simulink model "Torque_Control_ETR07"  (R2017b)
settings: Solver=FixedStepAuto  StartTime=0.0  StopTime=10.0  RelTol=1e-3
libraries: simulink x15
(part 2 of 5)

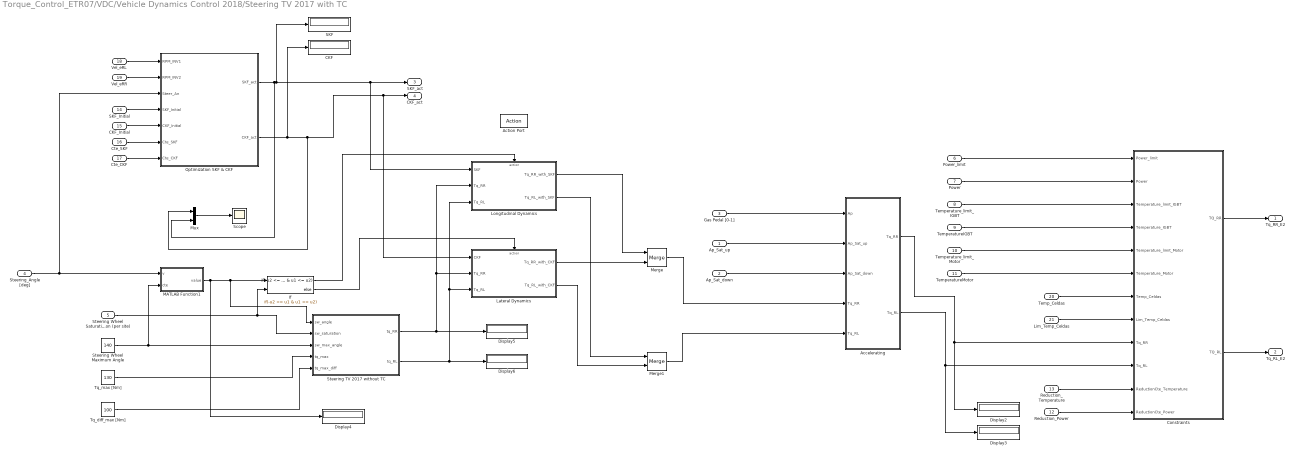
== system Torque_Control_ETR07/VDC/Vehicle Dynamics Control 2018/Steering TV 2017 with TC ==
  "Ap_Sat_up " : Inport
  Ap_Sat_down : Inport  Port=2
  Gas Pedal [0-1] : Inport  Port=3
  Steering_Angle [deg] : Inport  Port=4
  "Steering Wheel Saturation (per site) " : Inport  Port=5
  Power_limit : Inport  Port=6
  Power : Inport  Port=7
  Temperature_limit_IGBT : Inport  Port=8
  TemperatureIGBT : Inport  Port=9
  Temperature_limit_Motor : Inport  Port=10
  TemperatureMotor : Inport  Port=11
  Reduction_Power : Inport  Port=12
  Reduction_Temperature : Inport  Port=13
  SKF_Initial : Inport  Port=14
  CKF_Initial : Inport  Port=15
  Cte_SKF : Inport  Port=16
  Cte_CKF : Inport  Port=17
  Vel_eRL : Inport  Port=18
  Vel_eRR : Inport  Port=19
  Temp_Celdas : Inport  Port=20
  Lim_Temp_Celdas : Inport  Port=21
  Action Port : ActionPort  ActionType=elseif
  Accelerating : Subsystem
  CKF : Display
  Constraints : Subsystem
  Display{2..6} (5 alike) : Display
  If : If  NumInputs=2  IfExpression=-u2 <= u1 & u1 <= u2
  Lateral Dynamics : Subsystem  TreatAsAtomicUnit=on
  Longitudinal Dynamics : Subsystem  TreatAsAtomicUnit=on
  MATLAB Function1 : MATLAB Function  TreatAsAtomicUnit=on
  Merge : Merge
  Merge1 : Merge
  Mux : Mux  Inputs=2
  Optimization SKF & CKF : Subsystem
  SKF : Display
  Scope : Scope
  Steering TV 2017 without TC : MATLAB Function  TreatAsAtomicUnit=on
  Steering Wheel Maximum Angle : Constant  Value=140
  Tq_diff_max [Nm] : Constant  Value=100
  Tq_max [Nm] : Constant  Value=130
  Tq_RR_E2 : Outport
  Tq_RL_E2 : Outport  Port=2
  SKF_act : Outport  Port=3
  CKF_act : Outport  Port=4
  wires:
  Gas Pedal [0-1]/1 -> Accelerating/1(Ap)
  "Ap_Sat_up "/1 -> Accelerating/2("Ap_Sat_up ")
  Ap_Sat_down/1 -> Accelerating/3(Ap_Sat_down)
  Tq_max [Nm]/1 -> Steering TV 2017 without TC/4(tq_max)
  Tq_diff_max [Nm]/1 -> Steering TV 2017 without TC/5(tq_max_diff)
  Steering Wheel Maximum Angle/1 -> Steering TV 2017 without TC/3(sw_max_angle), MATLAB Function1/2(cte)
  "Steering Wheel Saturation (per site) "/1 -> If/2, Steering TV 2017 without TC/2(sw_saturation)
  Steering TV 2017 without TC/1(tq_RR) -> Display5/1, Longitudinal Dynamics/2(Tq_RR), Lateral Dynamics/2(Tq_RR)
  Steering TV 2017 without TC/2(tq_RL) -> Longitudinal Dynamics/3(Tq_RL), Lateral Dynamics/3(Tq_RL), Display6/1
  Power_limit/1 -> Constraints/1(Power_limit)
  Power/1 -> Constraints/2(Power)
  Temperature_limit_IGBT/1 -> Constraints/3(Temperature_limit_IGBT)
  TemperatureIGBT/1 -> Constraints/4(Temperature_IGBT)
  Reduction_Temperature/1 -> Constraints/11(ReductionCte_Temperature)
  Reduction_Power/1 -> Constraints/12(ReductionCte_Power)
  Constraints/1(TQ_RR) -> Tq_RR_E2/1
  Constraints/2(TQ_RL) -> Tq_RL_E2/1
  Accelerating/2(Tq_RL) -> Display3/1, Constraints/10(Tq_RL)
  Accelerating/1("Tq_RR ") -> Display2/1, Constraints/9(Tq_RR)
  MATLAB Function1/1(value) -> Display4/1, Steering TV 2017 without TC/1(sw_angle), If/1
  Temperature_limit_Motor/1 -> Constraints/5(Temperature_limit_Motor)
  TemperatureMotor/1 -> Constraints/6(Temperature_Motor)
  Optimization SKF & CKF/2(CKF_act) -> CKF/1, Mux/1, Lateral Dynamics/1(CKF), CKF_act/1
  SKF_Initial/1 -> Optimization SKF & CKF/4(SKF_Initial)
  Mux/1 -> Scope/1
  Cte_SKF/1 -> Optimization SKF & CKF/6(Cte_SKF)
  Vel_eRL/1 -> Optimization SKF & CKF/1(RPM_INV1)
  Vel_eRR/1 -> Optimization SKF & CKF/2(RPM_INV2)
  Optimization SKF & CKF/1(SKF_act) -> SKF_act/1, Longitudinal Dynamics/1(SKF), SKF/1, Mux/2
  Steering_Angle [deg]/1 -> MATLAB Function1/1(v), Optimization SKF & CKF/3(Steer_An)
  CKF_Initial/1 -> Optimization SKF & CKF/5(CKF_Initial)
  Cte_CKF/1 -> Optimization SKF & CKF/7(Cte_CKF)
  If/1 -> Longitudinal Dynamics/Action
  Lateral Dynamics/2(Tq_RL_with_CKF) -> Merge1/2
  If/2 -> Lateral Dynamics/Action
  Longitudinal Dynamics/2(Tq_RL_with_SKF) -> Merge1/1
  Longitudinal Dynamics/1(Tq_RR_with_SKF) -> Merge/1
  Lateral Dynamics/1(Tq_RR_with_CKF) -> Merge/2
  Merge/1 -> Accelerating/4(Tq_RR)
  Merge1/1 -> Accelerating/5("Tq_RL ")
  Temp_Celdas/1 -> Constraints/7(Temp_Celdas)
  Lim_Temp_Celdas/1 -> Constraints/8(Lim_Temp_Celdas)

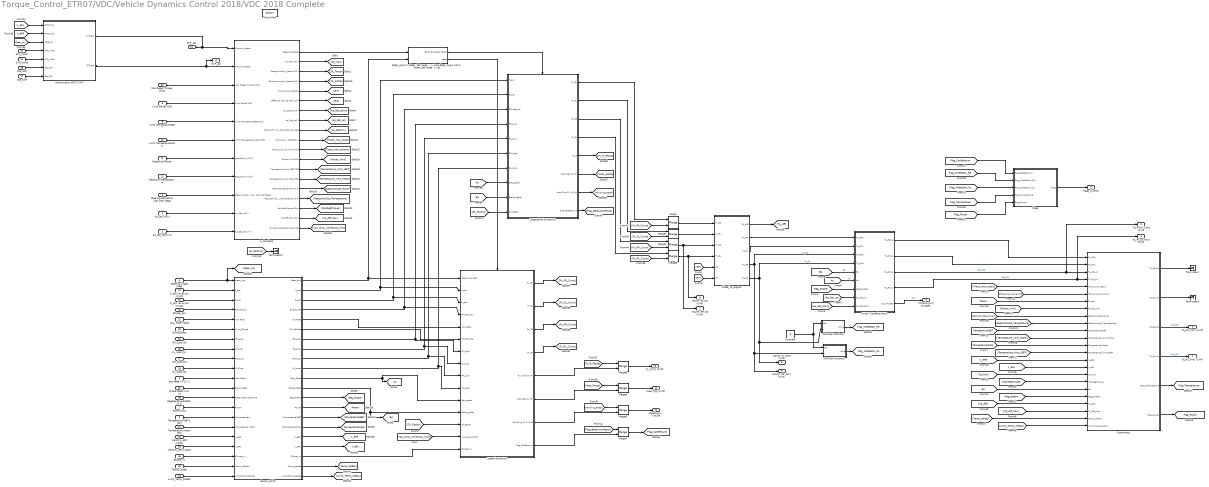
== system Torque_Control_ETR07/VDC/Vehicle Dynamics Control 2018/VDC 2018 Complete ==
  Ap_Sat_Up [-] : Inport
  Ap_Sat_Down [-] : Inport  Port=2
  Gas Pedal (0-1) [-] : Inport  Port=3
  Steering_Angle [deg] : Inport  Port=4
  Steering Saturation (per site) [deg] : Inport  Port=5
  Limit Power [kW] : Inport  Port=6
  Power [kW] : Inport  Port=7
  Limit TemperatureIGBT : Inport  Port=8
  Temperature IGBTs [ºC] : Inport  Port=9
  Limit TemperatureMotor : Inport  Port=10
  Temperature Motor [ºC] : Inport  Port=11
  Reduction Power : Inport  Port=12
  Reduction Temperature : Inport  Port=13
  SKF_Initial : Inport  Port=14
  CKF_Initial : Inport  Port=15
  Cte_SKF : Inport  Port=16
  Cte_CKF : Inport  Port=17
  Velocity_eRL [rad/s] : Inport  Port=18
  Velocity_eRR [rad/s] : Inport  Port=19
  Temp_Celdas : Inport  Port=20
  Limit_Temp_Celdas : Inport  Port=21
  F_acc (ax,ay,az) [m/s2] : Inport  Port=22
  R_acc (ax,ay,az) [m/s2] : Inport  Port=23
  Ellipse_acc : Inport  Port=24
  FR_Susp [N] : Inport  Port=25
  FL_Susp [N] : Inport  Port=26
  RR_Susp [N] : Inport  Port=27
  RL_Susp [N] : Inport  Port=28
  Regenerative Enable [0,1] : Inport  Port=29
  Max Regen Torque [Nm] : Inport  Port=30
  Brake Pedal (0-1) [-] : Inport  Port=31
  Yaw_Rate [rad/s] : Inport  Port=32
  Gyro_Ellipse : Inport  Port=33
  Ellipse_vx : Inport  Port=34
  Action Port : ActionPort  ActionType=then
  Constant : Constant  Value=0
  Constraints : Subsystem
  Driver / CarBehaviours : Subsystem
  Flags : Subsystem
  In_Numbers : Subsystem
  Lateral Dynamics : Subsystem  TreatAsAtomicUnit=on
  Longitudinal Dynamics : Subsystem  TreatAsAtomicUnit=on
  MATLAB Function1 : MATLAB Function  TreatAsAtomicUnit=on
  MATLAB Function2 : MATLAB Function  TreatAsAtomicUnit=on
  Merge{,1..7} (8 alike) : Merge
  Optimization SKF & CKF : Subsystem
  Sensor_DATA : Subsystem
  "Steer_ang is in Steer_Sat range ---> Long Steer_ang is not in Steer_Sat range -> Lat " : If  NumInputs=2  IfExpression=u2>=-u1&u2<=u1
  Terminator : Terminator
  Terminator1 : Terminator
  Terminator2 : Terminator
  Wheel_to_engine : Subsystem
  Tq_RR [Nm] (0,inf) : Outport
  Tq_RL [Nm] (0,inf) : Outport  Port=2
  Tq_RRwc [Nm] (0,inf) : Outport  Port=3
  Tq_RLwc [Nm] (0,inf) : Outport  Port=4
  MaxTq_RR [Nm] (0,inf) : Outport  Port=5
  MaxTq_RL [Nm] (0,inf) : Outport  Port=6
  MaxFx_RR [N] (0,inf) : Outport  Port=7
  MaxFx_RL [N] (0,inf) : Outport  Port=8
  Throttle [0-1] (0-100%) : Outport  Port=9
  Fy_R [N] (0,inf) : Outport  Port=10
  Mass [kg] (0,inf) : Outport  Port=11
  Handling [-] (-inf,inf) : Outport  Port=12
  Flags_[num5] : Outport  Port=13
  SKF_act : Outport  Port=14
  CKF_act : Outport  Port=15
  tag scope: Ap=global, Bp=global, Flag_CarBehavior=global, Flag_Power=global, Flag_Temperature=global, Flag_WheelSpin_RL=global, Flag_WheelSpin_RR=global, Power=global, Reg_enable=global, TemperatureIGBT=global, TemperatureMotor=global, V_eRL=global, V_eRR=global
  wires:
  "Steer_ang is in Steer_Sat range ---> Long Steer_ang is not in Steer_Sat range -> Lat "/1 -> Longitudinal Dynamics/Action
  "Steer_ang is in Steer_Sat range ---> Long Steer_ang is not in Steer_Sat range -> Lat "/2 -> Lateral Dynamics/Action
  Sensor_DATA/10(RL_susp) -> Lateral Dynamics/10(RL_susp), Longitudinal Dynamics/7(RL_susp)
  In_Numbers/3(Straight Kamm_Factor [0-2]) -> [SK_Factor]
  In_Numbers/1(Steer_Sat [deg]) -> "Steer_ang is in Steer_Sat range ---> Long Steer_ang is not in Steer_Sat range -> Lat "/1
  In_Numbers/2(Tq_Max [Nm]) -> [Tq_max]
  Sensor_DATA/11(Gas_Pedal) -> [Ap], Lateral Dynamics/11(Gas_pedal)
  In_Numbers/6(Effective Rolling Radius[m]) -> [Re]
  In_Numbers/5(Transmision_Ratio[-]) -> [RT]
  Sensor_DATA/9(RR_susp) -> Lateral Dynamics/9(RR_susp), Longitudinal Dynamics/6(RR_susp)
  In_Numbers/8(Ap_Sat_up[-]) -> [Ap_Sat_up]
  In_Numbers/7(Ap_Sat_down[-]) -> [Ap_Sat_down]
  Driver / CarBehaviours/3(Tq_RRout) -> Tq_RRwc [Nm] (0,inf)/1, Constraints/3(Tq_RR_wc)  "Teo_RR"
  Sensor_DATA/2(F_acc) -> Lateral Dynamics/2(F_acc), Longitudinal Dynamics/1(F_acc)
  Sensor_DATA/3(R_acc) -> Lateral Dynamics/3(R_acc), Longitudinal Dynamics/2(R_acc)
  Sensor_DATA/12(Brake_Pedal) -> [Bp], Lateral Dynamics/12(Brake_pedal)
  Sensor_DATA/8(FL_susp) -> Lateral Dynamics/8(FL_susp), Longitudinal Dynamics/5(FL_susp)
  Sensor_DATA/13(Reg_Enable) -> [Reg_enable]
  Sensor_DATA/7(FR_susp) -> Lateral Dynamics/7(FR_susp), Longitudinal Dynamics/4(FR_susp)
  Sensor_DATA/1(Steer_ang) -> "Steer_ang is in Steer_Sat range ---> Long Steer_ang is not in Steer_Sat range -> Lat "/2, Lateral Dynamics/1(Steering_Angle)
  Wheel_to_engine/5(Tq_RL) -> Driver / CarBehaviours/4("Tq_RLin "), MaxTq_RL [Nm] (0,inf)/1, MATLAB Function1/2(v)  "Tq_RL"
  [Trans_max_dynamic] -> Constraints/6(Trans_max_dynamic)
  [Power_limit] -> Constraints/8(Power_limit)
  In_Numbers/15(ReductionCte_Power (0-1)) -> [ReductionCte_Power]
  Driver / CarBehaviours/5(out_Throttle) -> Throttle [0-1] (0-100%)/1  "Out"
  Wheel_to_engine/4(Tq_RR) -> Driver / CarBehaviours/3(Tq_RRin), MaxTq_RR [Nm] (0,inf)/1, MATLAB Function2/2(v)  "Tq_RR"
  Wheel_to_engine/3(Tq_FL) -> Driver / CarBehaviours/2(Tq_FLin)
  In_Numbers/11(Trans_max_dynamic [Nm]) -> [Trans_max_dynamic]
  [Reg_enable] -> Driver / CarBehaviours/7(Reg_enable)
  [ReductionCte_Power] -> Constraints/9(ReductionCte_Power)
  [Ap_Sat_up] -> Driver / CarBehaviours/8(Ap_Sat_up)
  In_Numbers/10(Trans_max _static[Nm]) -> [Trans_max_static]
  [Ap] -> Driver / CarBehaviours/6(Ap)  "Ap"
  [Power] -> Constraints/7(Power)
  In_Numbers/12("Power limit [KW] ") -> [Power_limit]
  [Ap_Sat_down] -> Driver / CarBehaviours/9(Ap_Sat_down)
  Driver / CarBehaviours/4(Tq_RLout) -> Tq_RLwc [Nm] (0,inf)/1, Constraints/4("Tq_RL_wc ")  "Teo_RL"
  Driver / CarBehaviours/2("Tq_FLout ") -> Constraints/2(Tq_FLin)
  Steering_Angle [deg]/1 -> [Steer_An], Sensor_DATA/1(Steer_Ang)
  Wheel_to_engine/2(Tq_FR) -> Driver / CarBehaviours/1(Tq_FRin)
  Driver / CarBehaviours/1(Tq_FRout) -> Constraints/1(Tq_FRin)
  [Trans_max_static] -> Constraints/5("Trans_max_static ")
  [Temperature_limit_IGBT] -> Constraints/14(Temperature_limit_IGBT)
  [Bp] -> Constraints/19(Bp)
  Sensor_DATA/18(V_eRL) -> [V_eRL]
  In_Numbers/17(MaxRegTorque [Nm]) -> [MaxRegTorque]
  [TemperatureIGBT] -> Constraints/11(TemperatureIGBT)
  [Reg_enable] -> Constraints/20(Reg_enable)
  In_Numbers/9(Engine+Inverter Performance[-]) -> [ei_Perform]
  [Bp] -> Driver / CarBehaviours/5(Bp)  "Bp"
  [Tq_max] -> Constraints/17(Tq_max)
  RR_Susp [N]/1 -> Sensor_DATA/9(RR_Susp)
  Power [kW]/1 -> Sensor_DATA/14("Power ")
  Sensor_DATA/14(Power) -> [Power]
  Sensor_DATA/17("V_eRR ") -> [V_eRR]
  [V_eRR] -> Constraints/15(V_eRR)
  Regenerative Enable [0,1]/1 -> Sensor_DATA/13(Regenerative Enable)
  Brake Pedal (0-1) [-]/1 -> Sensor_DATA/12(Brake Pedal)
  [V_eRL] -> Constraints/16(V_eRL)
  In_Numbers/13(Temperature limit IGBT [ºC]) -> [Temperature_limit_IGBT]
  FL_Susp [N]/1 -> Sensor_DATA/8(FL_Susp)
  FR_Susp [N]/1 -> Sensor_DATA/7(FR_Susp)
  R_acc (ax,ay,az) [m/s2]/1 -> Sensor_DATA/3(R_Acc)
  F_acc (ax,ay,az) [m/s2]/1 -> Sensor_DATA/2("F_Acc ")
  RL_Susp [N]/1 -> Sensor_DATA/10(RL_Susp)
  Gas Pedal (0-1) [-]/1 -> Sensor_DATA/11(Gas Pedal)
  Temperature IGBTs [ºC]/1 -> Sensor_DATA/15(TemperatureIN)
  Velocity_eRR [rad/s]/1 -> Sensor_DATA/17(V_eRR)
  Velocity_eRL [rad/s]/1 -> Sensor_DATA/18("V_eRL ")
  Constraints/1(Tq_FRout) -> Terminator/1
  Constraints/2("Tq_FLout ") -> Terminator1/1
  In_Numbers/4(Cornering Kamm_Factor [0-2]) -> [CK_Factor]
  [Re] -> Wheel_to_engine/5(Re)
  [RT] -> Wheel_to_engine/6(RT)
  Merge3/1 -> MaxFx_RL [N] (0,inf)/1, Wheel_to_engine/4("Fx_RL ")
  Merge2/1 -> MaxFx_RR [N] (0,inf)/1, Wheel_to_engine/3("Fx_RR ")
  Merge1/1 -> Wheel_to_engine/2("Fx_FL ")
  Max Regen Torque [Nm]/1 -> In_Numbers/3(Max Regen Torque [Nm])
  Limit Power [kW]/1 -> In_Numbers/4(Limit Power [kW])
  Limit TemperatureIGBT/1 -> In_Numbers/5(Limit TemperatureIGBT [ºC])
  Reduction Power/1 -> In_Numbers/7(Reduction_P [0-1])
  [CK_Factor] -> Lateral Dynamics/13(CK_Factor)
  [SK_Factor] -> Longitudinal Dynamics/10(SK_Factor)
  Longitudinal Dynamics/1(Fx_FR) -> Merge/1
  Longitudinal Dynamics/2(Fx_FL) -> Merge1/1
  Longitudinal Dynamics/3("Fx_RR ") -> Merge2/1
  Longitudinal Dynamics/4("Fx_RL ") -> Merge3/1
  Merge/1 -> Wheel_to_engine/1("Fx_FR ")
  Steering Saturation (per site) [deg]/1 -> In_Numbers/9(Steering Saturation (per site) [deg])
  Ap_Sat_Up [-]/1 -> In_Numbers/10(Ap_Sat_Up [-])
  Ap_Sat_Down [-]/1 -> In_Numbers/11(Ap_Sat_Down [-])
  [MaxRegTorque] -> Constraints/18(MaxRegTorque)
  [ei_Perform] -> Terminator2/1
  Merge4/1 -> Mass [kg] (0,inf)/1
  Lateral Dynamics/6(" Mass [kg] (0,inf)") -> Merge4/2
  Lateral Dynamics/7(Handling [-] (-inf,inf)) -> Merge5/2
  Merge5/1 -> Handling [-] (-inf,inf)/1
  Merge6/1 -> Fy_R [N] (0,inf)/1
  Lateral Dynamics/5(Fy_R [N] (0,inf)) -> Merge6/2
  In_Numbers/16(ReductionCte_Temperature (0-1)) -> [ReductionCte_Temperature]
  Reduction Temperature/1 -> In_Numbers/8(Reduction_T [0-1])
  [ReductionCte_Temperature] -> Constraints/10(ReductionCte_Temperature)
  Constraints/3(Tq_RRout) -> Tq_RR [Nm] (0,inf)/1  "Out_RR"
  Constraints/4(Tq_RLout) -> Tq_RL [Nm] (0,inf)/1  "Out_RL"
  Temperature Motor [ºC]/1 -> Sensor_DATA/16(Temperature Motor)
  Sensor_DATA/15(TemperatureIGBT) -> [TemperatureIGBT]
  Sensor_DATA/16(TemperatureMotor) -> [TemperatureMotor]
  [TemperatureMotor] -> Constraints/13(TemperatureIMotor)
  [Temperature_limit_Motor] -> Constraints/12(TemperatureI_limit_Motor)
  In_Numbers/14(Temperature limit Motor [ºC]) -> [Temperature_limit_Motor]
  Limit TemperatureMotor/1 -> In_Numbers/6(Limit Temperature Motor [ºC])
  Merge7/1 -> [Flag_CarBehavior]
  Lateral Dynamics/8(Flag CarBehavior) -> Merge7/2
  MATLAB Function2/1(value) -> [Flag_WheelSpin_RL]
  MATLAB Function1/1(value) -> [Flag_WheelSpin_RR]
  Constant/1 -> MATLAB Function1/1(cte), MATLAB Function2/1(cte)
  Constraints/5(Flag_Temperature) -> [Flag_Temperature]
  Constraints/6(Flag_Power) -> [Flag_Power]
  Flags/1(Flags) -> Flags_[num5]/1
  [Flag_WheelSpin_RL] -> Flags/3(Flag_WheelSpin_RL)
  [Flag_WheelSpin_RR] -> Flags/2(Flag_WheelSpin_RR)
  [Flag_CarBehavior] -> Flags/1(Flag_CarBehavior)
  [Flag_Temperature] -> Flags/4(Flag_Temperature)
  [Flag_Power] -> Flags/5(Flag_Power)
  Optimization SKF & CKF/1(SKF_act) -> SKF_act/1, In_Numbers/1(S-Kamm_Factor)
  CKF_Initial/1 -> Optimization SKF & CKF/5(CKF_Initial)
  [Steer_An] -> Optimization SKF & CKF/3(Steer_An)
  [V_eRR] -> Optimization SKF & CKF/2(RPM_INV2)
  Cte_SKF/1 -> Optimization SKF & CKF/6(Cte_SKF)
  Cte_CKF/1 -> Optimization SKF & CKF/7(Cte_CKF)
  SKF_Initial/1 -> Optimization SKF & CKF/4(SKF_Initial)
  [V_eRL] -> Optimization SKF & CKF/1(RPM_INV1)
  Optimization SKF & CKF/2(CKF_act) -> CKF_act/1, In_Numbers/2(C-Kamm_Factor)
  Yaw_Rate [rad/s]/1 -> Sensor_DATA/5(Yaw Rate)
  Wheel_to_engine/1(Tq_diff) -> [Tq_diff]
  [Tq_diff] -> Constraints/21(Tq_diff)
  Sensor_DATA/5(YawRate) -> Lateral Dynamics/5(Yaw_Rate)
  Ellipse_acc/1 -> Sensor_DATA/4(Ellipse_acc)
  Gyro_Ellipse/1 -> Sensor_DATA/6(Gyro_Ellipse)
  Sensor_DATA/6(GyroEllipse) -> Lateral Dynamics/6(GyroEllipse)
  Sensor_DATA/4(Ellipse_Acc) -> Lateral Dynamics/4(Ellipse_Acc), Longitudinal Dynamics/3(Ellipse_Acc)
  In_Numbers/19(Yaw_error_correction_time [s]) -> [Yaw_error_correction_time]
  In_Numbers/18(Tq_diff_Max [Nm]) -> [Tq_diff_Max]
  [Yaw_error_correction_time] -> Lateral Dynamics/14(Yaw_error_/dt [s])
  [Ap] -> Longitudinal Dynamics/8(Gas_pedal)
  [Bp] -> Longitudinal Dynamics/9(Brake_pedal)
  Longitudinal Dynamics/6(Mass [kg] (0,inf)) -> [Mass_Recta]
  Longitudinal Dynamics/7(Handling [-] (-inf,inf)) -> [Handling_Recta]
  Longitudinal Dynamics/8(Flag CarBehavior) -> [Flag_BehaviourRecta]
  Longitudinal Dynamics/5(Fy_R) -> [Fy_R_Recta]
  [Fy_R_Recta] -> Merge6/1
  [Mass_Recta] -> Merge4/1
  [Handling_Recta] -> Merge5/1
  [Flag_BehaviourRecta] -> Merge7/1
  Lateral Dynamics/1(Fx_FR) -> [Fx_FR_Curva]
  Lateral Dynamics/2(Fx_FL) -> [Fx_FL_Curva]
  Lateral Dynamics/3("Fx_RR ") -> [Fx_RR_Curva]
  Lateral Dynamics/4("Fx_RL ") -> [Fx_RL_Curva]
  [Fx_FR_Curva] -> Merge/2
  [Fx_FL_Curva] -> Merge1/2
  [Fx_RR_Curva] -> Merge2/2
  [Fx_RL_Curva] -> Merge3/2
  Ellipse_vx/1 -> Sensor_DATA/19(Ellipse_vx)
  Sensor_DATA/19(Ellipse_Vx) -> Lateral Dynamics/15(Ellipse_Vx)
  [Tq_diff_Max] -> Constraints/22(Tq_diff_max)
  Temp_Celdas/1 -> Sensor_DATA/20(Temp_Celdas)
  Limit_Temp_Celdas/1 -> Sensor_DATA/21(Limit_Temp_Celdas)
  Sensor_DATA/20(Temp_celdas) -> [Temp_celdas]
  Sensor_DATA/21(Limit_Temp_celdas) -> [Limit_Temp_celdas]
  [Temp_celdas] -> Constraints/23(Temp_celdas)
  [Limit_Temp_celdas] -> Constraints/24(Limit_Temp_celdas)

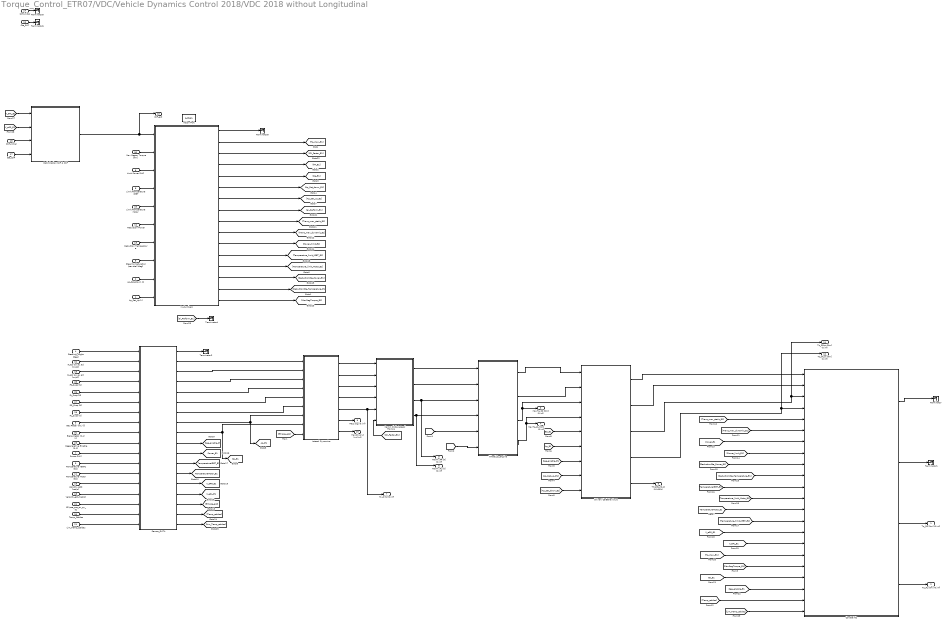
== system Torque_Control_ETR07/VDC/Vehicle Dynamics Control 2018/VDC 2018 without Longitudinal ==
  Ap_Sat_Up [-] : Inport
  Ap_Sat_Down [-] : Inport  Port=2
  Gas Pedal (0-1) [-] : Inport  Port=3
  Steering_Angle [deg] : Inport  Port=4
  Steering Saturation (per site) [deg] : Inport  Port=5
  Limit Power [kW] : Inport  Port=6
  Power [kW] : Inport  Port=7
  Limit Temperature IGBT : Inport  Port=8
  Temperature IGBTs [ºC] : Inport  Port=9
  Limit Temperature Motor : Inport  Port=10
  Temperature Motor [ºC] : Inport  Port=11
  Reduction Power : Inport  Port=12
  Reduction Temperature : Inport  Port=13
  SKF_initial : Inport  Port=14
  CKF_Initial : Inport  Port=15
  Cte_SKF : Inport  Port=16
  Cte_CKF : Inport  Port=17
  Velocity_eRL [rad/s] : Inport  Port=18
  Velocity_eRR [rad/s] : Inport  Port=19
  Temp_Celdas : Inport  Port=20
  Lim_Temp_Celdas : Inport  Port=21
  F_acc (ax,ay,az) [m/s2] : Inport  Port=22
  R_acc (ax,ay,az) [m/s2] : Inport  Port=23
  Ellipse_acc_ax_ay_az : Inport  Port=24
  FR_Susp [N] : Inport  Port=25
  FL_Susp [N] : Inport  Port=26
  RR_Susp [N] : Inport  Port=27
  RL_Susp [N] : Inport  Port=28
  Regenerative Enable [0,1] : Inport  Port=29
  Max Regen Torque [Nm] : Inport  Port=30
  Brake Pedal (0-1) [-] : Inport  Port=31
  Action Port : ActionPort  ActionType=elseif
  Constraints : Subsystem
  Driver / CarBehaviours : Subsystem
  In_Numbers : Subsystem
  Kamm Circle Lateral : Subsystem
  Lateral Dynamics : Subsystem
  Optimization SKF & CKF : Subsystem
  Sensor_DATA : Subsystem
  Terminator{,1..6} (7 alike) : Terminator
  Wheel_to_engine : Subsystem
  Tq_RR [Nm] (0,inf) : Outport
  Tq_RL [Nm] (0,inf) : Outport  Port=2
  MaxTq_RR [Nm] (0,inf) : Outport  Port=3
  MaxTq_RL [Nm] (0,inf) : Outport  Port=4
  MaxFx_RR [N] (0,inf) : Outport  Port=5
  MaxFx_RL [N] (0,inf) : Outport  Port=6
  Fy_R [N] (0,inf) : Outport  Port=7
  Throttle [0-1] (0-100%) : Outport  Port=8
  Mass [kg] (0,inf) : Outport  Port=9
  Handling [-] (-inf,inf) : Outport  Port=10
  Tq_RRwc [Nm] (0,inf) : Outport  Port=11
  Tq_RLwc [Nm] (0,inf) : Outport  Port=12
  CKF_act : Outport  Port=13
  tag scope: Ap_E1=global, Bp_E1=global, Power_E1=global, Reg_enable_E1=global, TemperatureIGBT_E1=global, TemperatureMotor_E1=global, V_eRL_E1=global, V_eRR_E1=global
  wires:
  Sensor_DATA/7(RL_susp) -> Lateral Dynamics/6(RL_susp)
  In_Numbers/2(Tq_Max [Nm]) -> [Tq_max_E1]
  Sensor_DATA/8(Gas_Pedal) -> [Ap_E1], Lateral Dynamics/7(Gas_pedal)
  In_Numbers/5(Effective Rolling Radius[m]) -> [Re_E1]
  In_Numbers/4(Transmision_Ratio[-]) -> [RT_E1]
  Sensor_DATA/6(RR_susp) -> Lateral Dynamics/5(RR_susp)
  In_Numbers/7(Ap_Sat_up[-]) -> [Ap_Sat_up_E1]
  In_Numbers/6(Ap_Sat_down[-]) -> [Ap_Sat_down_E1]
  Sensor_DATA/2(F_acc) -> Lateral Dynamics/1(F_acc)
  Sensor_DATA/3(R_acc) -> Lateral Dynamics/2(R_acc)
  Sensor_DATA/9(Brake_Pedal) -> [Bp_E1], Lateral Dynamics/8(Brake_pedal)
  Sensor_DATA/5(FL_susp) -> Lateral Dynamics/4(FL_susp)
  Sensor_DATA/10(Reg_Enable) -> [Reg_enable_E1]
  Sensor_DATA/4(FR_susp) -> Lateral Dynamics/3(FR_susp)
  Wheel_to_engine/4(Tq_RL) -> Driver / CarBehaviours/4("Tq_RLin "), MaxTq_RL [Nm] (0,inf)/1  "Tq_RL"
  In_Numbers/14(Reduction Power (0-1)) -> [ReductionCte_Power_E1]
  Wheel_to_engine/3(Tq_RR) -> MaxTq_RR [Nm] (0,inf)/1, Driver / CarBehaviours/3(Tq_RRin)  "Tq_RR"
  In_Numbers/10(Trans_max_dynamic [Nm]) -> [Trans_max_dynamic_E1]
  [Reg_enable_E1] -> Driver / CarBehaviours/7(Reg_enable)
  [Ap_Sat_up_E1] -> Driver / CarBehaviours/8(Ap_Sat_up)
  In_Numbers/9(Trans_max _static[Nm]) -> [Trans_max_static_E1]
  [Ap_E1] -> Driver / CarBehaviours/6(Ap)
  In_Numbers/11("Power limit [KW] ") -> [Power_limit_E1]
  [Ap_Sat_down_E1] -> Driver / CarBehaviours/9(Ap_Sat_down)
  Steering_Angle [deg]/1 -> Sensor_DATA/1(Steer_Ang)
  Sensor_DATA/15(V_eRL) -> [V_eRL_E1]
  In_Numbers/16(MaxRegTorque [Nm]) -> [MaxRegTorque_E1]
  In_Numbers/8(Engine+Inverter Performance[-]) -> [ei_Perform_E1]
  [Bp_E1] -> Driver / CarBehaviours/5(Bp)
  Sensor_DATA/12(Temperature IGBT) -> [TemperatureIGBT_E1]
  RR_Susp [N]/1 -> Sensor_DATA/6(RR_Susp)
  Power [kW]/1 -> Sensor_DATA/11("Power ")
  Sensor_DATA/11(Power) -> [Power_E1]
  Sensor_DATA/14("V_eRR ") -> [V_eRR_E1]
  Regenerative Enable [0,1]/1 -> Sensor_DATA/10(Regenerative Enable)
  Brake Pedal (0-1) [-]/1 -> Sensor_DATA/9(Brake Pedal)
  In_Numbers/12(Temperature limit IGBT [ºC]) -> [Temperature_limit_IGBT_E1]
  FL_Susp [N]/1 -> Sensor_DATA/5(FL_Susp)
  FR_Susp [N]/1 -> Sensor_DATA/4(FR_Susp)
  R_acc (ax,ay,az) [m/s2]/1 -> Sensor_DATA/3(R_Acc)
  F_acc (ax,ay,az) [m/s2]/1 -> Sensor_DATA/2("F_Acc ")
  RL_Susp [N]/1 -> Sensor_DATA/7(RL_Susp)
  Gas Pedal (0-1) [-]/1 -> Sensor_DATA/8(Gas Pedal)
  Temperature IGBTs [ºC]/1 -> Sensor_DATA/12(TemperatureIGBT)
  Velocity_eRR [rad/s]/1 -> Sensor_DATA/14(V_eRR)
  Velocity_eRL [rad/s]/1 -> Sensor_DATA/15("V_eRL ")
  Max Regen Torque [Nm]/1 -> In_Numbers/2(Max Regen Torque [Nm])
  Limit Power [kW]/1 -> In_Numbers/3(Limit Power [kW])
  Limit Temperature IGBT/1 -> In_Numbers/4(Limit Temperature IGBT [ºC])
  Reduction Power/1 -> In_Numbers/6(Reduction Power [0-1])
  In_Numbers/3(Cornering Kamm_Factor [0-2]) -> [CK_Factor_E1]
  [Re_E1] -> Wheel_to_engine/5(Re)
  [RT_E1] -> Wheel_to_engine/6(RT)
  Ap_Sat_Up [-]/1 -> In_Numbers/10(Ap_Sat_Up [-])
  Ap_Sat_Down [-]/1 -> In_Numbers/9(Ap_Sat_Down [-])
  Steering Saturation (per site) [deg]/1 -> In_Numbers/8(Steering Saturation (per site) [deg])
  [CK_Factor_E1] -> Kamm Circle Lateral/6(CK_Factor)
  Kamm Circle Lateral/1(Fx_FR) -> Wheel_to_engine/1("Fx_FR ")
  Kamm Circle Lateral/2(Fx_FL) -> Wheel_to_engine/2("Fx_FL ")
  Kamm Circle Lateral/3("Fx_RR ") -> MaxFx_RR [N] (0,inf)/1, Wheel_to_engine/3("Fx_RR ")
  Kamm Circle Lateral/4("Fx_RL ") -> MaxFx_RL [N] (0,inf)/1, Wheel_to_engine/4("Fx_RL ")
  Sensor_DATA/1(Steer_ang) -> Terminator2/1
  Lateral Dynamics/1(N_FR) -> Kamm Circle Lateral/1("N_FR ")
  Lateral Dynamics/2("N_FL ") -> Kamm Circle Lateral/2(N_FL)
  Lateral Dynamics/3("N_RR ") -> Kamm Circle Lateral/3(N_RR)
  Lateral Dynamics/4(N_RL) -> Kamm Circle Lateral/4(N_RL)
  Driver / CarBehaviours/5(out_Throttle) -> Throttle [0-1] (0-100%)/1  "Out"
  [ei_Perform_E1] -> Terminator4/1
  In_Numbers/1(Steer_Sat [deg]) -> Terminator5/1
  Lateral Dynamics/6(Mass [kg] (0,inf)) -> Mass [kg] (0,inf)/1
  Lateral Dynamics/7(Handling [-] (-inf,inf)) -> Handling [-] (-inf,inf)/1
  In_Numbers/15(Reduction Temperature (0-1)) -> [ReductionCte_Temperature_E1]
  Reduction Temperature/1 -> In_Numbers/7(Reduction Temperature [0-1])
  Driver / CarBehaviours/3(Tq_RRout) -> Tq_RRwc [Nm] (0,inf)/1, Constraints/3(Tq_RR_wc)  "Teo_RR"
  [Trans_max_dynamic_E1] -> Constraints/6(Trans_max_dynamic)
  [Power_limit_E1] -> Constraints/8(Power_limit)
  [ReductionCte_Power_E1] -> Constraints/9(ReductionCte_Power)
  [Power_E1] -> Constraints/7(Power)
  Driver / CarBehaviours/4(Tq_RLout) -> Tq_RLwc [Nm] (0,inf)/1, Constraints/4("Tq_RL_wc ")  "Teo_RL"
  Driver / CarBehaviours/2("Tq_FLout ") -> Constraints/2(Tq_FLin)
  Driver / CarBehaviours/1(Tq_FRout) -> Constraints/1(Tq_FRin)
  [Trans_max_static_E1] -> Constraints/5("Trans_max_static ")
  [Temperature_limit_IGBT_E1] -> Constraints/14(Temperature_limit_IGBT)
  [Bp_E1] -> Constraints/19(Bp)
  [TemperatureIGBT_E1] -> Constraints/11(TemperatureIGBT)
  [Reg_enable_E1] -> Constraints/20(Reg_enable)
  [Tq_max_E1] -> Constraints/17(Tq_max)
  [V_eRR_E1] -> Constraints/15(V_eRR)
  [V_eRL_E1] -> Constraints/16(V_eRL)
  Constraints/1(Tq_FRout) -> Terminator/1
  Constraints/2("Tq_FLout ") -> Terminator1/1
  [MaxRegTorque_E1] -> Constraints/18(MaxRegTorque)
  [ReductionCte_Temperature_E1] -> Constraints/10(ReductionCte_Temperature)
  [TemperatureMotor_E1] -> Constraints/13(TemperatureIMotor)
  [Temperature_limit_Motor_E1] -> Constraints/12(TemperatureI_limit_Motor)
  Limit Temperature Motor/1 -> In_Numbers/5(Limit Temperature Motor [ºC])
  In_Numbers/13(Temperature limit Motor [ºC]) -> [Temperature_limit_Motor_E1]
  Temperature Motor [ºC]/1 -> Sensor_DATA/13(TemperatureMotor)
  Sensor_DATA/13(Temperature Motor) -> [TemperatureMotor_E1]
  [V_eRR_E1] -> Optimization SKF & CKF/2(RPM_INV2)
  CKF_Initial/1 -> Optimization SKF & CKF/3(CKF_Initial)
  Cte_CKF/1 -> Optimization SKF & CKF/4(Cte_CKF)
  Optimization SKF & CKF/1(CKF_act) -> CKF_act/1, In_Numbers/1(C-Kamm_Factor)
  [V_eRL_E1] -> Optimization SKF & CKF/1(RPM_INV1)
  Constraints/3(Tq_RRout) -> Tq_RR [Nm] (0,inf)/1  "Out_RR"
  Constraints/4(Tq_RLout) -> Tq_RL [Nm] (0,inf)/1  "Out_RL"
  Ellipse_acc_ax_ay_az/1 -> Sensor_DATA/16(Ellipse_acc_ax_ay_az)
  Sensor_DATA/16(Ellipse_acc) -> [Ellipse_acc]
  Lateral Dynamics/5(Fy_R) -> Kamm Circle Lateral/5(Fy), Fy_R [N] (0,inf)/1
  [Ellipse_acc] -> Lateral Dynamics/9(Ellipse_acc)
  Temp_Celdas/1 -> Sensor_DATA/17(Temp_Celdas)
  Lim_Temp_Celdas/1 -> Sensor_DATA/18(Lim_Temp_Celdas)
  Sensor_DATA/17(temp_celdas) -> [Temp_celdas]
  Sensor_DATA/18(Lim_temp_celdas) -> [Lim_Temp_celdas]
  [Temp_celdas] -> Constraints/21(Temp_celdas)
  [Lim_Temp_celdas] -> Constraints/22(Limit_Temp_Celdas)
  SKF_initial/1 -> Terminator3/1
  Cte_SKF/1 -> Terminator6/1
  Wheel_to_engine/2(Tq_FL) -> Driver / CarBehaviours/2(Tq_FLin)
  Wheel_to_engine/1(Tq_FR) -> Driver / CarBehaviours/1(Tq_FRin)

== system Torque_Control_ETR07/VDC/WORKSHOP_MODE_RESTRICTIONS/BYPASS ==
  In1 : Inport
  In2 : Inport  Port=2
  Action Port : ActionPort  ActionType=else
  Out1 : Outport
  Out2 : Outport  Port=2
  wires:
  In1/1 -> Out1/1
  In2/1 -> Out2/1

== system Torque_Control_ETR07/VDC/WORKSHOP_MODE_RESTRICTIONS/Torque_Reduction  ==
  In1 : Inport
  In2 : Inport  Port=2
  Action Port : ActionPort  ActionType=then
  Constant : Constant  Value=15
  Divide : Product  Inputs=*/
  Divide1 : Product  Inputs=*/
  Saturation : Saturate  UpperLimit=10  LowerLimit=-10
  Saturation1 : Saturate  UpperLimit=10  LowerLimit=-10
  Out1 : Outport
  Out2 : Outport  Port=2
  wires:
  Saturation/1 -> Out1/1
  Saturation1/1 -> Out2/1
  In1/1 -> Divide/1
  Divide/1 -> Saturation/1
  In2/1 -> Divide1/1
  Divide1/1 -> Saturation1/1
  Constant/1 -> Divide1/2, Divide/2

== system Torque_Control_ETR07/Accumulator Power/PowerLimitDetection/OK_OrLatch/Latched Error ==
  Action Port : ActionPort  ActionType=then
  Constant : Constant
  "Out " : Outport
  wires:
  Constant/1 -> "Out "/1

== system Torque_Control_ETR07/Accumulator Power/PowerLimitDetection/OK_OrLatch/OK ==
  Action Port : ActionPort  ActionType=else
  Constant : Constant  Value=0
  "Out " : Outport
  wires:
  Constant/1 -> "Out "/1

== system Torque_Control_ETR07/VDC/Regeneration_Enable/Not-Braking/Low_Threshold ==
  Action Port : ActionPort  ActionType=else
  TEMP_LIMIT_LOWER : Constant  Value=45
  Out1 : Outport
  wires:
  TEMP_LIMIT_LOWER/1 -> Out1/1

== system Torque_Control_ETR07/VDC/Regeneration_Enable/Not-Braking/Temp_LIMIT ==
  Action Port : ActionPort  ActionType=then
  TEMP_LIMIT : Constant  Value=0
  Out1 : Outport
  wires:
  TEMP_LIMIT/1 -> Out1/1

== system Torque_Control_ETR07/VDC/Regeneration_Enable/Not-Braking/Temp_OK ==
  Action Port : ActionPort  ActionType=else
  TEMP_LIMIT : Constant
  Out1 : Outport
  wires:
  TEMP_LIMIT/1 -> Out1/1

== system Torque_Control_ETR07/VDC/Regeneration_Enable/Not-Braking/Upper_Threshold ==
  Action Port : ActionPort  ActionType=then
  TEMP_LIMIT_UPPER : Constant  Value=50
  Out1 : Outport
  wires:
  TEMP_LIMIT_UPPER/1 -> Out1/1

== system Torque_Control_ETR07/VDC/Vehicle Dynamics Control 2018/Rigid Axle/Accelerating ==
  Ap : Inport
  "Ap_Sat_up " : Inport  Port=2
  Ap_Sat_down : Inport  Port=3
  Tq_RR : Inport  Port=4
  "Tq_RL " : Inport  Port=5
  "Accelerator behaviour " : MATLAB Function  TreatAsAtomicUnit=on
  Product : Product
  Product1 : Product
  "Tq_RR " : Outport
  Tq_RL : Outport  Port=2
  wires:
  Ap_Sat_down/1 -> "Accelerator behaviour "/3(Ap_Sat_down)
  Product/1 -> Tq_RL/1
  "Accelerator behaviour "/1(throttle) -> Product/1, Product1/1
  "Ap_Sat_up "/1 -> "Accelerator behaviour "/2(Ap_Sat_up)
  Ap/1 -> "Accelerator behaviour "/1(Ap)
  Tq_RR/1 -> Product1/2
  "Tq_RL "/1 -> Product/2
  Product1/1 -> "Tq_RR "/1

== system Torque_Control_ETR07/VDC/Vehicle Dynamics Control 2018/Steering TV 2017 with TC/Accelerating ==
  Ap : Inport
  "Ap_Sat_up " : Inport  Port=2
  Ap_Sat_down : Inport  Port=3
  Tq_RR : Inport  Port=4
  "Tq_RL " : Inport  Port=5
  "Accelerator behaviour " : MATLAB Function  TreatAsAtomicUnit=on
  Product : Product
  Product1 : Product
  "Tq_RR " : Outport
  Tq_RL : Outport  Port=2
  wires:
  Ap_Sat_down/1 -> "Accelerator behaviour "/3(Ap_Sat_down)
  Product/1 -> Tq_RL/1
  "Accelerator behaviour "/1(throttle) -> Product/1, Product1/1
  "Ap_Sat_up "/1 -> "Accelerator behaviour "/2(Ap_Sat_up)
  Ap/1 -> "Accelerator behaviour "/1(Ap)
  Tq_RR/1 -> Product1/2
  "Tq_RL "/1 -> Product/2
  Product1/1 -> "Tq_RR "/1

== system Torque_Control_ETR07/VDC/Vehicle Dynamics Control 2018/Steering TV 2017 with TC/Constraints ==
  note: Considero de la misma gravedad,
      | la limitacion por potencia que por temperatura
  Power_limit : Inport
  Power : Inport  Port=2
  Temperature_limit_IGBT : Inport  Port=3
  Temperature_IGBT : Inport  Port=4
  Temperature_limit_Motor : Inport  Port=5
  Temperature_Motor : Inport  Port=6
  Temp_Celdas : Inport  Port=7
  Lim_Temp_Celdas : Inport  Port=8
  Tq_RR : Inport  Port=9
  Tq_RL : Inport  Port=10
  ReductionCte_Temperature : Inport  Port=11
  ReductionCte_Power : Inport  Port=12
  "Control de Potencia " : Subsystem  TreatAsAtomicUnit=on
  Control de Temperatura : Subsystem  TreatAsAtomicUnit=on
  If : If  NumInputs=8  IfExpression=u4 >= u3 | u6 >= u5 | u7>=u8  ElseIfExpressions=u2 >= u1
  Merge : Merge  Inputs=3
  Merge1 : Merge  Inputs=3
  else : Subsystem  TreatAsAtomicUnit=on
  TQ_RR : Outport
  TQ_RL : Outport  Port=2
  wires:
  ReductionCte_Power/1 -> "Control de Potencia "/3(ReductionCte)
  Power_limit/1 -> If/1
  Temperature_limit_IGBT/1 -> If/3
  ReductionCte_Temperature/1 -> Control de Temperatura/3(ReductionCte)
  Power/1 -> If/2
  "Control de Potencia "/1(Tq_RR_out) -> Merge/1
  "Control de Potencia "/2(Tq_RL_out) -> Merge1/1
  else/2(Tq_RL_out) -> Merge1/3
  If/1 -> Control de Temperatura/Action
  Tq_RR/1 -> else/1(Tq_RR), Control de Temperatura/1(Tq_RR), "Control de Potencia "/1(Tq_RR)
  Tq_RL/1 -> Control de Temperatura/2(Tq_RL), "Control de Potencia "/2(Tq_RL), else/2(Tq_RL)
  If/2 -> "Control de Potencia "/Action
  If/3 -> else/Action
  Control de Temperatura/1(Tq_RR_out) -> Merge/2
  else/1(Tq_RR_out) -> Merge/3
  Control de Temperatura/2(Tq_RL_out) -> Merge1/2
  Temperature_limit_Motor/1 -> If/5
  Temperature_Motor/1 -> If/6
  Merge/1 -> TQ_RR/1
  Merge1/1 -> TQ_RL/1
  Temperature_IGBT/1 -> If/4
  Temp_Celdas/1 -> If/7
  Lim_Temp_Celdas/1 -> If/8

== system Torque_Control_ETR07/VDC/Vehicle Dynamics Control 2018/Steering TV 2017 with TC/Lateral Dynamics ==
  CKF : Inport
  Tq_RR : Inport  Port=2
  Tq_RL : Inport  Port=3
  Action Port : ActionPort  ActionType=else
  Product : Product
  Product1 : Product
  Tq_RR_with_CKF : Outport
  Tq_RL_with_CKF : Outport  Port=2
  wires:
  Product1/1 -> Tq_RL_with_CKF/1
  Tq_RR/1 -> Product/1
  Tq_RL/1 -> Product1/1
  CKF/1 -> Product/2, Product1/2
  Product/1 -> Tq_RR_with_CKF/1

== system Torque_Control_ETR07/VDC/Vehicle Dynamics Control 2018/Steering TV 2017 with TC/Longitudinal Dynamics ==
  SKF : Inport
  Tq_RR : Inport  Port=2
  Tq_RL : Inport  Port=3
  Action Port : ActionPort  ActionType=then
  Product : Product
  Product1 : Product
  Tq_RR_with_SKF : Outport
  Tq_RL_with_SKF : Outport  Port=2
  wires:
  Tq_RR/1 -> Product/1
  Tq_RL/1 -> Product1/1
  SKF/1 -> Product/2, Product1/2
  Product/1 -> Tq_RR_with_SKF/1
  Product1/1 -> Tq_RL_with_SKF/1

== system Torque_Control_ETR07/VDC/Vehicle Dynamics Control 2018/Steering TV 2017 with TC/Optimization SKF & CKF ==
  RPM_INV1 : Inport
  RPM_INV2 : Inport  Port=2
  Steer_An : Inport  Port=3
  SKF_Initial : Inport  Port=4
  CKF_Initial : Inport  Port=5
  Cte_SKF : Inport  Port=6
  Cte_CKF : Inport  Port=7
  CKF_prev : DataStoreRead  DataStoreName=B
  Constant : Constant  Value=0
  Data Store Memory : DataStoreMemory  ReadBeforeWriteMsg=warning  WriteAfterWriteMsg=warning  WriteAfterReadMsg=warning  ShowAdditionalParam=off
  Data Store Memory1 : DataStoreMemory  DataStoreName=B  ReadBeforeWriteMsg=warning  WriteAfterWriteMsg=warning  WriteAfterReadMsg=warning  ShowAdditionalParam=off
  Data Store Write : DataStoreWrite
  Data Store Write1 : DataStoreWrite  DataStoreName=B
  Derivative : Derivative
  Display : Display
  MATLAB Function : MATLAB Function  TreatAsAtomicUnit=on
  Mux : Mux  Inputs=3
  "SKF_prev " : DataStoreRead
  Saturation : Saturate  UpperLimit=6000  LowerLimit=0
  Scope{,1,3..5} (5 alike) : Scope
  Scope2 : Scope  NumInputPorts=2
  Scope7 : Scope  NumInputPorts=3
  Signal Generator : SignalGenerator  WaveForm=square  Units=rad/sec
  Sine Wave : Sin  SampleTime=0
  "Subsystem " : Subsystem
  Switch : Switch  Threshold=900
  SKF_act : Outport
  CKF_act : Outport  Port=2
  wires:
  SKF_Initial/1 -> "Subsystem "/3(SKF_Initial)
  "Subsystem "/1("SKF_act ") -> SKF_act/1, Data Store Write/1  "SKF"
  Derivative/1 -> Scope2/2, Scope7/2, Display/1, "Subsystem "/2(Derivative), Switch/1, Switch/2, Saturation/1  "alpha"
  "Subsystem "/2(CKF_act) -> CKF_act/1, Scope7/1, Data Store Write1/1  "CKF"
  Cte_CKF/1 -> "Subsystem "/8(Cte_CKF)
  Steer_An/1 -> "Subsystem "/1(Steer_An)
  CKF_Initial/1 -> "Subsystem "/5("CKF_Initial ")
  Cte_SKF/1 -> "Subsystem "/7(Cte_SKF)
  MATLAB Function/1(RPM) -> Scope7/3, Scope1/1, Derivative/1  "w (rad/s)"
  Mux/1 -> Scope/1
  Saturation/1 -> Mux/2
  Switch/1 -> Mux/3
  Constant/1 -> Switch/3
  RPM_INV1/1 -> MATLAB Function/1(RPM_INV1), Mux/1
  "SKF_prev "/1 -> "Subsystem "/4(SKF_prev)
  Signal Generator/1 -> Scope4/1
  Sine Wave/1 -> Scope5/1
  CKF_prev/1 -> "Subsystem "/6("CKF_prev ")
  RPM_INV2/1 -> Scope3/1, MATLAB Function/2(RPM_INV2), Scope2/1

== system Torque_Control_ETR07/VDC/Vehicle Dynamics Control 2018/VDC 2018 Complete/Constraints ==
  Tq_FRin : Inport
  Tq_FLin : Inport  Port=2
  Tq_RR_wc : Inport  Port=3
  "Tq_RL_wc " : Inport  Port=4
  "Trans_max_static " : Inport  Port=5
  Trans_max_dynamic : Inport  Port=6
  Power : Inport  Port=7
  Power_limit : Inport  Port=8
  ReductionCte_Power : Inport  Port=9
  ReductionCte_Temperature : Inport  Port=10
  TemperatureIGBT : Inport  Port=11
  TemperatureI_limit_Motor : Inport  Port=12
  TemperatureIMotor : Inport  Port=13
  Temperature_limit_IGBT : Inport  Port=14
  V_eRR : Inport  Port=15
  V_eRL : Inport  Port=16
  Tq_max : Inport  Port=17
  MaxRegTorque : Inport  Port=18
  Bp : Inport  Port=19
  Reg_enable : Inport  Port=20
  Tq_diff : Inport  Port=21
  Tq_diff_max : Inport  Port=22
  Temp_celdas : Inport  Port=23
  Limit_Temp_celdas : Inport  Port=24
  Acelerating and braking without Regenerative : Subsystem  TreatAsAtomicUnit=on
  Braking with Regenerative : Subsystem  TreatAsAtomicUnit=on
  Constant : Constant  Value=0
  Constant1 : Constant  Value=0
  If : If  NumInputs=2  IfExpression=u2 == 1 & u1 > 0
  Merge1 : Merge
  Merge2 : Merge
  Tq_FRout : Outport
  "Tq_FLout " : Outport  Port=2
  Tq_RRout : Outport  Port=3
  Tq_RLout : Outport  Port=4
  Flag_Temperature : Outport  Port=5
  Flag_Power : Outport  Port=6
  wires:
  Constant1/1 -> "Tq_FLout "/1
  Constant/1 -> Tq_FRout/1
  Tq_RR_wc/1 -> Braking with Regenerative/2(Tq_RR_wc), Acelerating and braking without Regenerative/16(Tq_RR)
  "Tq_RL_wc "/1 -> Braking with Regenerative/3(Tq_RL_wc), Acelerating and braking without Regenerative/17(Tq_RL)
  Tq_max/1 -> Acelerating and braking without Regenerative/1(Tq_max)
  V_eRL/1 -> Acelerating and braking without Regenerative/3(V_eRL)
  Trans_max_dynamic/1 -> Acelerating and braking without Regenerative/4(Trans_max_dynamic)
  "Trans_max_static "/1 -> Acelerating and braking without Regenerative/5(Trans_max_static)
  Merge2/1 -> Tq_RLout/1
  Merge1/1 -> Tq_RRout/1
  Bp/1 -> If/1
  Reg_enable/1 -> If/2
  V_eRR/1 -> Acelerating and braking without Regenerative/2(V_eRR)
  If/1 -> Braking with Regenerative/Action
  If/2 -> Acelerating and braking without Regenerative/Action
  MaxRegTorque/1 -> Braking with Regenerative/1(MaxRegTorque)
  Tq_FRin/1 -> Acelerating and braking without Regenerative/14(Tq_FR)
  Tq_FLin/1 -> Acelerating and braking without Regenerative/15(Tq_FL)
  ReductionCte_Temperature/1 -> Acelerating and braking without Regenerative/13(ReductionCte_Temperature)
  ReductionCte_Power/1 -> Acelerating and braking without Regenerative/12(ReductionCte_Power)
  TemperatureIGBT/1 -> Acelerating and braking without Regenerative/9(TemperatureIGBT)
  Temperature_limit_IGBT/1 -> Acelerating and braking without Regenerative/8(Temperature_limit_IGBT)
  Power/1 -> Acelerating and braking without Regenerative/7(Power)
  Power_limit/1 -> Acelerating and braking without Regenerative/6(Power_limit)
  Acelerating and braking without Regenerative/2(TQ_RL) -> Merge2/1
  Acelerating and braking without Regenerative/1(TQ_RR) -> Merge1/1
  Braking with Regenerative/1(TQ_RR) -> Merge1/2
  Braking with Regenerative/2(TQ_RL) -> Merge2/2
  TemperatureI_limit_Motor/1 -> Acelerating and braking without Regenerative/10(TemperatureI_limit_Motor)
  TemperatureIMotor/1 -> Acelerating and braking without Regenerative/11(TemperatureMotor)
  Acelerating and braking without Regenerative/4(Flag_Power) -> Flag_Power/1
  Acelerating and braking without Regenerative/3(Flag_Temperature) -> Flag_Temperature/1
  Tq_diff/1 -> Acelerating and braking without Regenerative/18(Tq_diff)
  Tq_diff_max/1 -> Acelerating and braking without Regenerative/19(Tq_diff_max)
  Temp_celdas/1 -> Acelerating and braking without Regenerative/20(Temp_celdas)
  Limit_Temp_celdas/1 -> Acelerating and braking without Regenerative/21(Limit_Temp_celdas)

== system Torque_Control_ETR07/VDC/Vehicle Dynamics Control 2018/VDC 2018 Complete/Driver // CarBehaviours ==
  Tq_FRin : Inport
  Tq_FLin : Inport  Port=2
  Tq_RRin : Inport  Port=3
  "Tq_RLin " : Inport  Port=4
  Bp : Inport  Port=5
  Ap : Inport  Port=6
  Reg_enable : Inport  Port=7
  Ap_Sat_up : Inport  Port=8
  Ap_Sat_down : Inport  Port=9
  Accelerating : Subsystem  TreatAsAtomicUnit=on
  "Accelerator behaviour " : MATLAB Function  TreatAsAtomicUnit=on
  Braking Conditions : If  NumInputs=3  IfExpression=u1>0 & u2<0.1 & u3==1  ElseIfExpressions=u1>0 & u2<0.1 & u3==0, u1<0.1 & u2<0.1
  Constant : Constant  Value=0
  Constant1 : Constant  Value=0
  Inertia Braking : Subsystem  TreatAsAtomicUnit=on
  Mech_Braking : Subsystem  TreatAsAtomicUnit=on
  Merge : Merge  Inputs=4
  Merge1 : Merge  Inputs=4
  Regenerative+Mech Braking : Subsystem  TreatAsAtomicUnit=on
  Terminator : Terminator
  Terminator1 : Terminator
  Tq_FRout : Outport
  "Tq_FLout " : Outport  Port=2
  Tq_RRout : Outport  Port=3
  Tq_RLout : Outport  Port=4
  out_Throttle : Outport  Port=5
  wires:
  Constant1/1 -> "Tq_FLout "/1
  Constant/1 -> Tq_FRout/1
  Tq_FLin/1 -> Terminator1/1
  Tq_FRin/1 -> Terminator/1
  Merge/1 -> Tq_RRout/1
  Merge1/1 -> Tq_RLout/1
  Bp/1 -> Braking Conditions/1
  Regenerative+Mech Braking/1("Tq_RR ") -> Merge/1
  Mech_Braking/1("Tq_RR ") -> Merge/2
  Inertia Braking/1("Tq_RR ") -> Merge/3
  Accelerating/1("Tq_RR ") -> Merge/4
  Regenerative+Mech Braking/2(Tq_RL) -> Merge1/1
  Mech_Braking/2(Tq_RL) -> Merge1/2
  Inertia Braking/2(Tq_RL) -> Merge1/3
  Accelerating/2(Tq_RL) -> Merge1/4
  Braking Conditions/1 -> Regenerative+Mech Braking/Action
  Braking Conditions/2 -> Mech_Braking/Action
  Braking Conditions/3 -> Inertia Braking/Action
  Braking Conditions/4 -> Accelerating/Action
  Tq_RRin/1 -> Accelerating/2(Tq_RR), Regenerative+Mech Braking/1(RegTq_RR)
  "Tq_RLin "/1 -> Accelerating/3("Tq_RL "), Regenerative+Mech Braking/2(RegTq_RL)
  Reg_enable/1 -> Braking Conditions/3
  Accelerating/3(Out_Throttle) -> out_Throttle/1
  "Accelerator behaviour "/1(throttle) -> Accelerating/1(Throttle), Braking Conditions/2
  Ap/1 -> "Accelerator behaviour "/1(Ap)
  Ap_Sat_up/1 -> "Accelerator behaviour "/2(Ap_Sat_up)
  Ap_Sat_down/1 -> "Accelerator behaviour "/3(Ap_Sat_down)

== system Torque_Control_ETR07/VDC/Vehicle Dynamics Control 2018/VDC 2018 Complete/Flags ==
  Flag_CarBehavior : Inport
  Flag_WheelSpin_RR : Inport  Port=2
  Flag_WheelSpin_RL : Inport  Port=3
  Flag_Temperature : Inport  Port=4
  Flag_Power : Inport  Port=5
  Mux : Mux  Inputs=5
  Flags : Outport
  wires:
  Mux/1 -> Flags/1
  Flag_CarBehavior/1 -> Mux/1
  Flag_WheelSpin_RR/1 -> Mux/2
  Flag_WheelSpin_RL/1 -> Mux/3
  Flag_Temperature/1 -> Mux/4
  Flag_Power/1 -> Mux/5

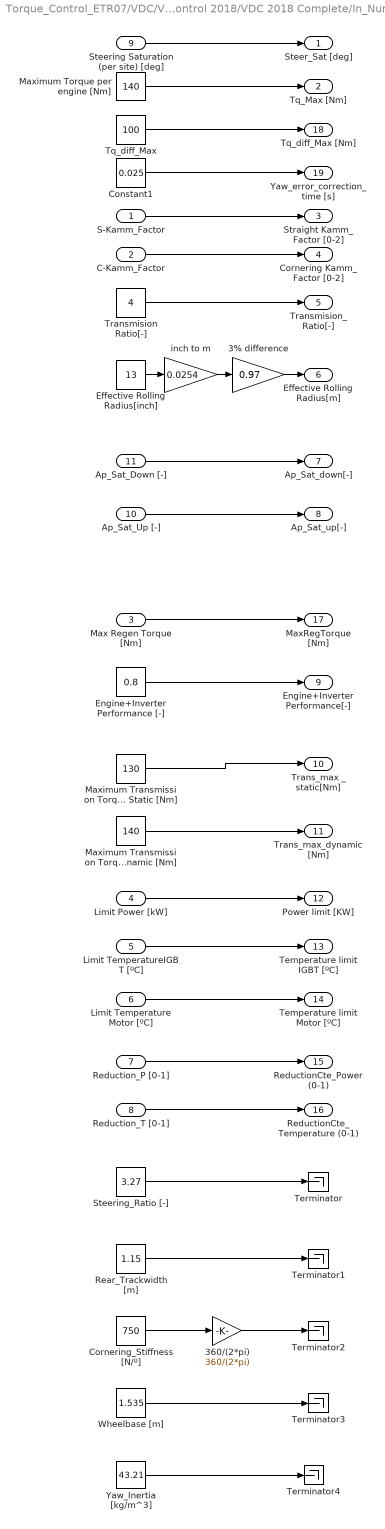
== system Torque_Control_ETR07/VDC/Vehicle Dynamics Control 2018/VDC 2018 Complete/In_Numbers ==
  S-Kamm_Factor : Inport
  C-Kamm_Factor : Inport  Port=2
  Max Regen Torque [Nm] : Inport  Port=3
  Limit Power [kW] : Inport  Port=4
  Limit TemperatureIGBT [ºC] : Inport  Port=5
  Limit Temperature Motor [ºC] : Inport  Port=6
  Reduction_P [0-1] : Inport  Port=7
  Reduction_T [0-1] : Inport  Port=8
  Steering Saturation (per site) [deg] : Inport  Port=9
  Ap_Sat_Up [-] : Inport  Port=10
  Ap_Sat_Down [-] : Inport  Port=11
  3% difference : Gain  Gain=0.97
  360/(2*pi) : Gain  Gain=360/(2*pi)
  Constant1 : Constant  Value=0.025
  Cornering_Stiffness [N/º] : Constant  Value=750
  Effective Rolling Radius[inch] : Constant  Value=13
  Engine+Inverter Performance [-] : Constant  Value=0.8
  Maximum Torque per engine [Nm] : Constant  Value=140
  Maximum Transmission Torque Dynamic [Nm] : Constant  Value=140
  Maximum Transmission Torque Static [Nm] : Constant  Value=130
  "Rear_Trackwidth [m] " : Constant  Value=1.15
  Steering_Ratio [-] : Constant  Value=3.27
  Terminator{,1..4} (5 alike) : Terminator
  Tq_diff_Max : Constant  Value=100
  Transmision Ratio[-] : Constant  Value=4
  Wheelbase [m] : Constant  Value=1.535
  Yaw_Inertia [kg/m^3] : Constant  Value=43.21  VectorParams1D=off  SampleTime=-1
  inch to m : Gain  Gain=0.0254
  Steer_Sat [deg] : Outport
  Tq_Max [Nm] : Outport  Port=2
  Straight Kamm_Factor [0-2] : Outport  Port=3
  Cornering Kamm_Factor [0-2] : Outport  Port=4
  Transmision_Ratio[-] : Outport  Port=5
  Effective Rolling Radius[m] : Outport  Port=6
  Ap_Sat_down[-] : Outport  Port=7
  Ap_Sat_up[-] : Outport  Port=8
  Engine+Inverter Performance[-] : Outport  Port=9
  Trans_max _static[Nm] : Outport  Port=10
  Trans_max_dynamic [Nm] : Outport  Port=11
  "Power limit [KW] " : Outport  Port=12
  Temperature limit IGBT [ºC] : Outport  Port=13
  Temperature limit Motor [ºC] : Outport  Port=14
  ReductionCte_Power (0-1) : Outport  Port=15
  ReductionCte_Temperature (0-1) : Outport  Port=16
  MaxRegTorque [Nm] : Outport  Port=17
  Tq_diff_Max [Nm] : Outport  Port=18  VectorParamsAs1DForOutWhenUnconnected=on
  Yaw_error_correction_time [s] : Outport  Port=19  VectorParamsAs1DForOutWhenUnconnected=on
  wires:
  Maximum Torque per engine [Nm]/1 -> Tq_Max [Nm]/1
  Transmision Ratio[-]/1 -> Transmision_Ratio[-]/1
  Effective Rolling Radius[inch]/1 -> inch to m/1
  Maximum Transmission Torque Static [Nm]/1 -> Trans_max _static[Nm]/1
  Maximum Transmission Torque Dynamic [Nm]/1 -> Trans_max_dynamic [Nm]/1
  inch to m/1 -> 3% difference/1
  3% difference/1 -> Effective Rolling Radius[m]/1
  Engine+Inverter Performance [-]/1 -> Engine+Inverter Performance[-]/1
  S-Kamm_Factor/1 -> Straight Kamm_Factor [0-2]/1
  Max Regen Torque [Nm]/1 -> MaxRegTorque [Nm]/1
  Limit Power [kW]/1 -> "Power limit [KW] "/1
  Limit TemperatureIGBT [ºC]/1 -> Temperature limit IGBT [ºC]/1
  Reduction_P [0-1]/1 -> ReductionCte_Power (0-1)/1
  C-Kamm_Factor/1 -> Cornering Kamm_Factor [0-2]/1
  Steering Saturation (per site) [deg]/1 -> Steer_Sat [deg]/1
  Ap_Sat_Up [-]/1 -> Ap_Sat_up[-]/1
  Ap_Sat_Down [-]/1 -> Ap_Sat_down[-]/1
  Reduction_T [0-1]/1 -> ReductionCte_Temperature (0-1)/1
  Limit Temperature Motor [ºC]/1 -> Temperature limit Motor [ºC]/1
  Steering_Ratio [-]/1 -> Terminator/1
  "Rear_Trackwidth [m] "/1 -> Terminator1/1
  Cornering_Stiffness [N/º]/1 -> 360/(2*pi)/1
  Wheelbase [m]/1 -> Terminator3/1
  360/(2*pi)/1 -> Terminator2/1
  Yaw_Inertia [kg/m^3]/1 -> Terminator4/1
  Tq_diff_Max/1 -> Tq_diff_Max [Nm]/1
  Constant1/1 -> Yaw_error_correction_time [s]/1

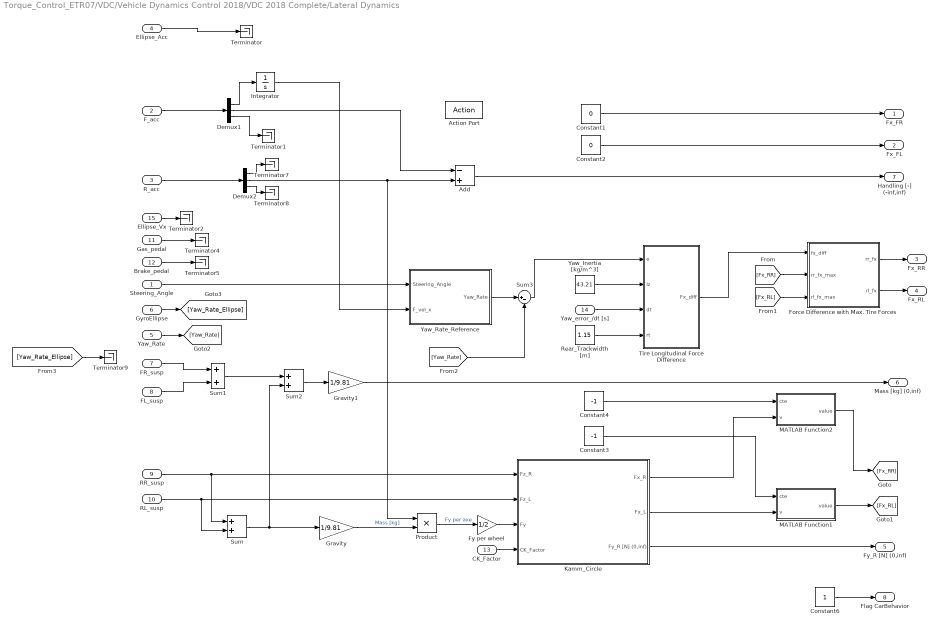
== system Torque_Control_ETR07/VDC/Vehicle Dynamics Control 2018/VDC 2018 Complete/Lateral Dynamics ==
  Steering_Angle : Inport
  F_acc : Inport  Port=2
  R_acc : Inport  Port=3
  Ellipse_Acc : Inport  Port=4
  Yaw_Rate : Inport  Port=5
  GyroEllipse : Inport  Port=6
  FR_susp : Inport  Port=7
  FL_susp : Inport  Port=8
  RR_susp : Inport  Port=9
  RL_susp : Inport  Port=10
  Gas_pedal : Inport  Port=11
  Brake_pedal : Inport  Port=12
  CK_Factor : Inport  Port=13
  Yaw_error_/dt [s] : Inport  Port=14
  Ellipse_Vx : Inport  Port=15
  Action Port : ActionPort  ActionType=else
  Add : Sum  Inputs=-+
  Constant1 : Constant  Value=0
  Constant2 : Constant  Value=0
  Constant3 : Constant  Value=-1
  Constant4 : Constant  Value=-1
  Constant6 : Constant
  Demux1 : Demux  Outputs=3
  Demux2 : Demux  Outputs=3
  Force Difference with Max. Tire Forces : MATLAB Function  TreatAsAtomicUnit=on
  Fy per wheel : Gain  Gain=1/2
  Gravity : Gain  Gain=1/9.81
  Gravity1 : Gain  Gain=1/9.81
  Integrator : Integrator
  Kamm_Circle : Subsystem
  MATLAB Function1 : MATLAB Function  TreatAsAtomicUnit=on
  MATLAB Function2 : MATLAB Function  TreatAsAtomicUnit=on
  Product : Product
  "Rear_Trackwidth [m] " : Constant  Value=1.15
  Sum : Sum
  Sum1 : Sum
  Sum2 : Sum
  Sum3 : Sum  Inputs=|+-
  Terminator{,1..2,4..5,7..9} (8 alike) : Terminator
  Tire Longitudinal Force Difference : Subsystem
  Yaw_Inertia [kg/m^3] : Constant  Value=43.21  VectorParams1D=off  SampleTime=-1
  Yaw_Rate_Reference : Subsystem
  Fx_FR : Outport
  Fx_FL : Outport  Port=2
  "Fx_RR " : Outport  Port=3
  "Fx_RL " : Outport  Port=4
  Fy_R [N] (0,inf) : Outport  Port=5
  " Mass [kg] (0,inf)" : Outport  Port=6
  Handling [-] (-inf,inf) : Outport  Port=7
  Flag CarBehavior : Outport  Port=8
  wires:
  Constant6/1 -> Flag CarBehavior/1
  Yaw_error_/dt [s]/1 -> Tire Longitudinal Force Difference/3(dt)
  "Rear_Trackwidth [m] "/1 -> Tire Longitudinal Force Difference/4(rt)
  Yaw_Inertia [kg/m^3]/1 -> Tire Longitudinal Force Difference/2(Iz)
  Tire Longitudinal Force Difference/1(Fx_diff) -> Force Difference with Max. Tire Forces/1(fx_diff)
  Sum3/1 -> Tire Longitudinal Force Difference/1(e)
  Yaw_Rate/1 -> [Yaw_Rate]
  Yaw_Rate_Reference/1(Yaw_Rate) -> Sum3/1
  [Fx_RL] -> Force Difference with Max. Tire Forces/3(rl_fx_max)
  [Fx_RR] -> Force Difference with Max. Tire Forces/2(rr_fx_max)
  MATLAB Function1/1(value) -> [Fx_RL]
  MATLAB Function2/1(value) -> [Fx_RR]
  Force Difference with Max. Tire Forces/1(rr_fx) -> "Fx_RR "/1
  Force Difference with Max. Tire Forces/2(rl_fx) -> "Fx_RL "/1
  Steering_Angle/1 -> Yaw_Rate_Reference/1(Steering_Angle)
  Kamm_Circle/1(Fx_R) -> MATLAB Function2/2(v)
  RL_susp/1 -> Kamm_Circle/2(Fz_L), Sum/2
  RR_susp/1 -> Kamm_Circle/1(Fz_R), Sum/1
  FL_susp/1 -> Sum1/2
  FR_susp/1 -> Sum1/1
  Demux1/1 -> Integrator/1
  Kamm_Circle/2(Fx_L) -> MATLAB Function1/2(v)
  Constant4/1 -> MATLAB Function2/1(cte)
  Constant3/1 -> MATLAB Function1/1(cte)
  Demux1/2 -> Add/1
  Add/1 -> Handling [-] (-inf,inf)/1
  Demux1/3 -> Terminator1/1
  F_acc/1 -> Demux1/1
  Gravity1/1 -> " Mass [kg] (0,inf)"/1
  Sum2/1 -> Gravity1/1
  Sum1/1 -> Sum2/1
  Gravity/1 -> Product/2  "Mass [kg]"
  Sum/1 -> Gravity/1, Sum2/2
  Kamm_Circle/3(Fy_R [N] (0,inf)) -> Fy_R [N] (0,inf)/1
  CK_Factor/1 -> Kamm_Circle/4(CK_Factor)
  Fy per wheel/1 -> Kamm_Circle/3(Fy)
  Constant2/1 -> Fx_FL/1
  Constant1/1 -> Fx_FR/1
  Product/1 -> Fy per wheel/1  "Fy per axe"
  Brake_pedal/1 -> Terminator5/1
  Gas_pedal/1 -> Terminator4/1
  GyroEllipse/1 -> [Yaw_Rate_Ellipse]
  [Yaw_Rate] -> Sum3/2
  Demux2/2 -> Product/1, Add/2
  Demux2/3 -> Terminator8/1
  Demux2/1 -> Terminator7/1
  R_acc/1 -> Demux2/1
  [Yaw_Rate_Ellipse] -> Terminator9/1
  Ellipse_Vx/1 -> Terminator2/1
  Integrator/1 -> Yaw_Rate_Reference/2(F_vel_x)
  Ellipse_Acc/1 -> Terminator/1
